simulink model "Lab_04_GMSK"  (Simulink 10.2)
settings: Solver=VariableStepAuto  StartTime=0.0  StopTime=10.0  RelTol=1e-3
libraries: commdigbbndcpm2 x7, commrandsrc3 x1, commutil2 x1
settings Model: Creator=Newtr  LastModifiedBy=Lenovo
settings DataIOCC: SaveFormat=Dataset  SignalLoggingSaveFormat=Dataset  ReturnWorkspaceOutputs=on
settings OptimizationCC: LifeSpan=auto
settings DebuggingCC: UnderspecifiedInitializationDetection=Simplified  MergeDetectMultiDrivingBlocksExec=error  FcnCallInpInsideContextMsg=error  SFUnexpectedBacktrackingDiag=error  SFNoUnconditionalDefaultTransitionDiag=error  SFExecutionAtInitializationDiag=warning  ArithmeticOperatorsInVariantConditions=error
settings HardwareCC: ProdBitPerPointer=64  ProdBitPerSizeT=64  ProdBitPerPtrDiffT=64  ProdLargestAtomicFloat=Float  ProdIntDivRoundTo=Zero  ProdEndianess=LittleEndian  ProdWordSize=64  ProdHWDeviceType=Intel->x86-64 (Windows64)
settings ModelReferenceCC: PropagateSignalLabelsOutOfModel=on
settings SFSimCC: SimUseLocalCustomCode=on  CustomCodeUndefinedFunction=FilterOut
settings RTWCC: RTWUseLocalCustomCode=on
settings CodeAppCC: StateflowObjectComments=off
settings GRTTargetCC: TargetLangStandard=C99 (ISO)  CombineOutputUpdateFcns=on  GRTInterface=off
settings ConfigComp: CovMetricSettings=dwe  CovSaveCumulativeToWorkspaceVar=off  CovSaveSingleToWorkspaceVar=off  CovExternalEMLEnable=on

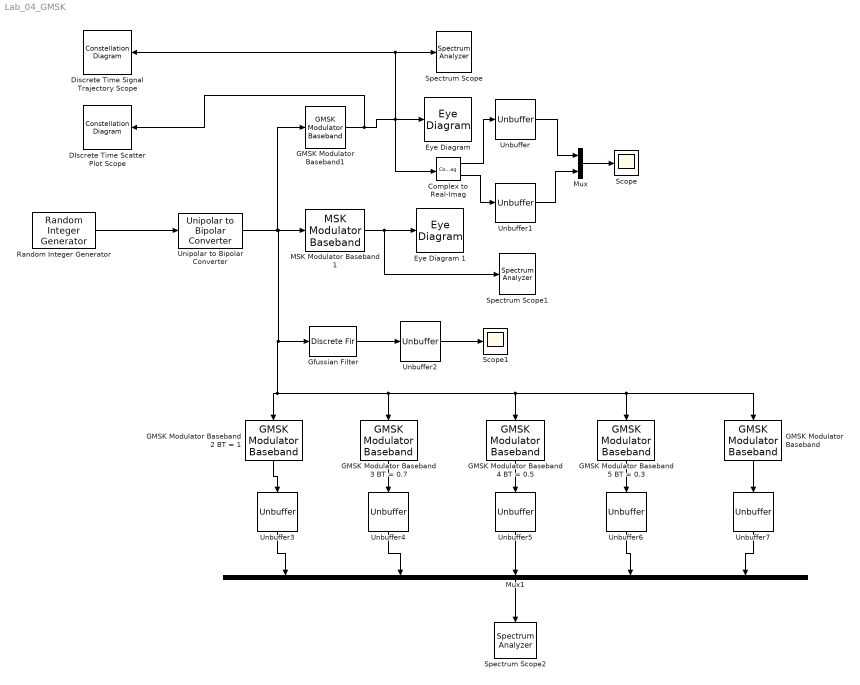
== system Lab_04_GMSK ==
  Complex to Real-Imag : ComplexToRealImag
  DIscrete Time Scatter Plot Scope : ConstellationDiagram
  Discrete Time Signal Trajectory Scope : ConstellationDiagram
  "Eye Diagram " : EyeDiagram
  Eye Diagram 1 : EyeDiagram
  GMSK Modulator Baseband : commdigbbndcpm2/GMSK Modulator Baseband  inputType=Integer  BT=.3  pulseLength=4  preHistory=1  phaseOffset=0  samplesPerSymbol=8  RateOptions=Enforce single-rate processing  outDataType=double
      settings: SourceProductBaseCode=CM
  GMSK Modulator Baseband 2 BT = 1 : commdigbbndcpm2/GMSK Modulator Baseband  inputType=Integer  BT=.3  pulseLength=4  preHistory=1  phaseOffset=0  samplesPerSymbol=8  RateOptions=Enforce single-rate processing  outDataType=double
      settings: SourceProductBaseCode=CM
  GMSK Modulator Baseband 3 BT = 0.7 : commdigbbndcpm2/GMSK Modulator Baseband  inputType=Integer  BT=.3  pulseLength=4  preHistory=1  phaseOffset=0  samplesPerSymbol=8  RateOptions=Enforce single-rate processing  outDataType=double
      settings: SourceProductBaseCode=CM
  GMSK Modulator Baseband 4 BT = 0.5 : commdigbbndcpm2/GMSK Modulator Baseband  inputType=Integer  BT=.3  pulseLength=4  preHistory=1  phaseOffset=0  samplesPerSymbol=8  RateOptions=Enforce single-rate processing  outDataType=double
      settings: SourceProductBaseCode=CM
  GMSK Modulator Baseband 5 BT = 0.3 : commdigbbndcpm2/GMSK Modulator Baseband  inputType=Integer  BT=.3  pulseLength=4  preHistory=1  phaseOffset=0  samplesPerSymbol=8  RateOptions=Enforce single-rate processing  outDataType=double
      settings: SourceProductBaseCode=CM
  GMSK Modulator Baseband1 : commdigbbndcpm2/GMSK Modulator Baseband  inputType=Integer  BT=.3  pulseLength=4  preHistory=1  phaseOffset=0  samplesPerSymbol=8  RateOptions=Enforce single-rate processing  outDataType=double
      settings: SourceProductBaseCode=CM
  Gfussian Filter : DiscreteFir  Coefficients=0.3  InputProcessing=Columns as channels (frame based)
  MSK Modulator Baseband 1 : commdigbbndcpm2/MSK Modulator Baseband  inputType=Integer  phaseOffset=0  samplesPerSymbol=8  RateOptions=Enforce single-rate processing  outDataType=double
      settings: SourceProductBaseCode=CM
  Mux : Mux  Inputs=2
  Mux1 : Mux  Inputs=5
  Random Integer Generator : commrandsrc3/Random Integer Generator  SetSize=2  SeedSource=Parameter  Seed=500  SampleTime=1/270000  SamplesPerFrame=1  OutputDataType=uint32  SimulateUsing=Interpreted execution
  Scope : Scope
  Scope1 : Scope
  Spectrum Scope : SpectrumAnalyzer
  Spectrum Scope1 : SpectrumAnalyzer
  Spectrum Scope2 : SpectrumAnalyzer
  Unbuffer{,1..7} (8 alike) : Unbuffer
  Unipolar to Bipolar Converter : commutil2/Unipolar to Bipolar Converter  M=2  polarity=Positive  dataType=double
  wires:
  Random Integer Generator/1 -> Unipolar to Bipolar Converter/1
  Unipolar to Bipolar Converter/1 -> GMSK Modulator Baseband1/1, Gfussian Filter/1, GMSK Modulator Baseband 2 BT = 1/1, GMSK Modulator Baseband 3 BT = 0.7/1, GMSK Modulator Baseband 4 BT = 0.5/1, GMSK Modulator Baseband 5 BT = 0.3/1, GMSK Modulator Baseband/1, MSK Modulator Baseband 1/1
  Gfussian Filter/1 -> Unbuffer2/1
  Unbuffer2/1 -> Scope1/1
  MSK Modulator Baseband 1/1 -> Spectrum Scope1/1, Eye Diagram 1/1
  GMSK Modulator Baseband1/1 -> DIscrete Time Scatter Plot Scope/1, Complex to Real-Imag/1, Spectrum Scope/1, Discrete Time Signal Trajectory Scope/1, "Eye Diagram "/1
  Complex to Real-Imag/1 -> Unbuffer/1
  Complex to Real-Imag/2 -> Unbuffer1/1
  Unbuffer/1 -> Mux/1
  Unbuffer1/1 -> Mux/2
  Mux/1 -> Scope/1
  GMSK Modulator Baseband 2 BT = 1/1 -> Unbuffer3/1
  GMSK Modulator Baseband 3 BT = 0.7/1 -> Unbuffer4/1
  GMSK Modulator Baseband 4 BT = 0.5/1 -> Unbuffer5/1
  GMSK Modulator Baseband 5 BT = 0.3/1 -> Unbuffer6/1
  GMSK Modulator Baseband/1 -> Unbuffer7/1
  Unbuffer3/1 -> Mux1/1
  Unbuffer4/1 -> Mux1/2
  Unbuffer5/1 -> Mux1/3
  Unbuffer6/1 -> Mux1/4
  Unbuffer7/1 -> Mux1/5
  Mux1/1 -> Spectrum Scope2/1
